simulink model "Inverse_v1"  (R2022a)
settings: Solver=VariableStepAuto  StartTime=0.0  StopTime=10.0  RelTol=1e-3
settings Model: Creator=maximilian  LastModifiedBy=maximilian

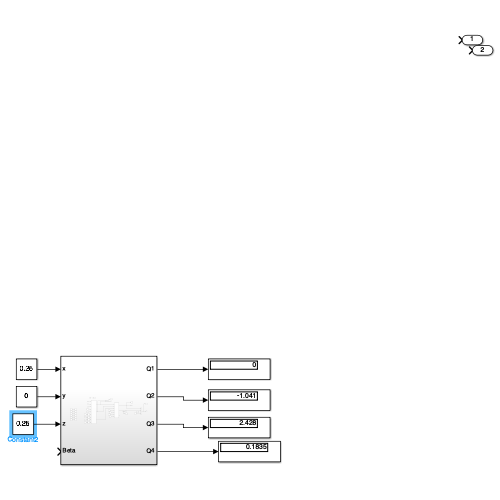
[thumbnail: Simulink's stored preview of the top-level diagram]
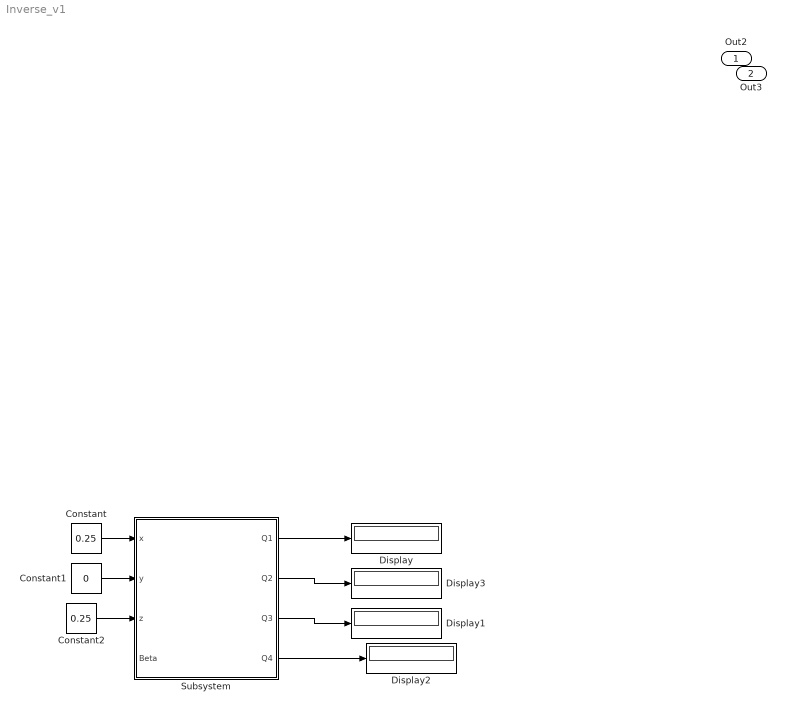
== system Inverse_v1 ==
  Constant : Constant  Value=0.25
  Constant1 : Constant  Value=0
  Constant2 : Constant  Value=0.25
  Display{,1..3} (4 alike) : Display
  Subsystem : Subsystem
  Out2 : Outport
  Out3 : Outport  Port=2
  wires:
  Constant2/1 -> Subsystem/3(z)
  Constant/1 -> Subsystem/1(x)
  Constant1/1 -> Subsystem/2(y)
  Subsystem/1(Q1) -> Display/1
  Subsystem/2(Q2) -> Display3/1
  Subsystem/3(Q3) -> Display1/1
  Subsystem/4(Q4) -> Display2/1

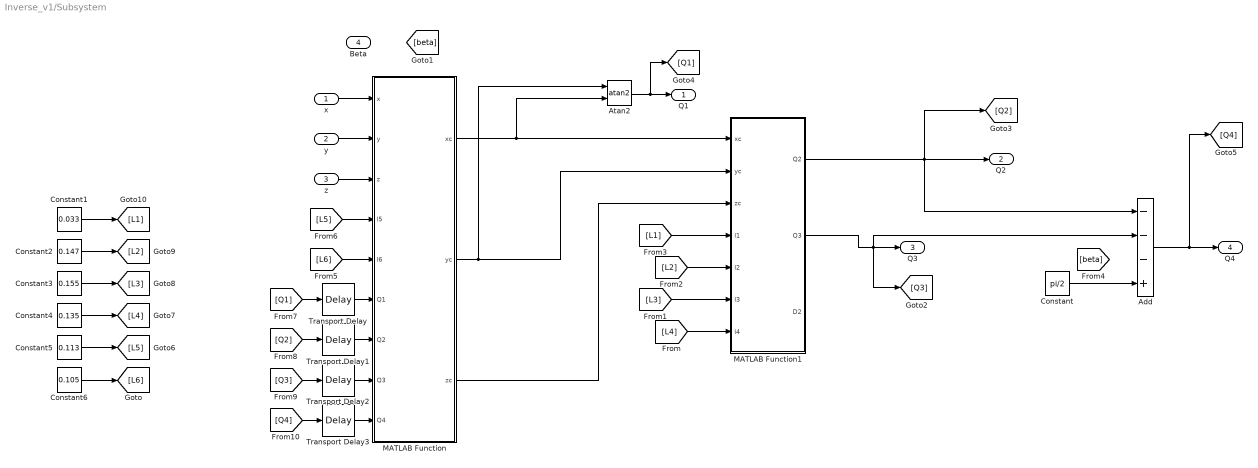
== system Inverse_v1/Subsystem ==
  x : Inport
  y : Inport  Port=2
  z : Inport  Port=3
  Beta : Inport  Port=4
  Add : Sum  Inputs=---+
  Atan2 : Trigonometry  Operator=atan2
  Constant : Constant  Value=pi/2
  Constant1 : Constant  Value=0.033
  Constant2 : Constant  Value=0.147
  Constant3 : Constant  Value=0.155
  Constant4 : Constant  Value=0.135
  Constant5 : Constant  Value=0.113
  Constant6 : Constant  Value=0.105
  MATLAB Function : MATLAB Function  TreatAsAtomicUnit=on
  MATLAB Function1 : MATLAB Function  TreatAsAtomicUnit=on
  Transport Delay{,1..3} (4 alike) : TransportDelay
  Q1 : Outport
  Q2 : Outport  Port=2
  Q3 : Outport  Port=3
  Q4 : Outport  Port=4
  wires:
  MATLAB Function/3(zc) -> MATLAB Function1/3(zc)
  Constant2/1 -> [L2]
  MATLAB Function/2(yc) -> Atan2/1, MATLAB Function1/2(yc)
  [L2] -> MATLAB Function1/5(l2)
  MATLAB Function1/2(Q3) -> Add/2, Q3/1, [Q3]
  Constant/1 -> Add/4
  [L3] -> MATLAB Function1/6(l3)
  [Q1] -> Transport Delay/1
  [Q4] -> Transport Delay3/1
  Transport Delay2/1 -> MATLAB Function/8(Q3)
  Transport Delay/1 -> MATLAB Function/6(Q1)
  [L1] -> MATLAB Function1/4(l1)
  [L5] -> MATLAB Function/4(l5)
  Transport Delay1/1 -> MATLAB Function/7(Q2)
  Constant1/1 -> [L1]
  Add/1 -> [Q4], Q4/1
  Atan2/1 -> Q1/1, [Q1]
  z/1 -> MATLAB Function/3(z)
  [Q3] -> Transport Delay2/1
  MATLAB Function/1(xc) -> MATLAB Function1/1(xc), Atan2/2
  x/1 -> MATLAB Function/1(x)
  [L4] -> MATLAB Function1/7(l4)
  MATLAB Function1/1(Q2) -> Add/1, Q2/1, [Q2]
  Transport Delay3/1 -> MATLAB Function/9(Q4)
  y/1 -> MATLAB Function/2(y)
  [L6] -> MATLAB Function/5(l6)
  [Q2] -> Transport Delay1/1
  Constant4/1 -> [L4]
  Constant6/1 -> [L6]
  Constant3/1 -> [L3]
  Constant5/1 -> [L5]

== matlab function Inverse_v1/Subsystem/MATLAB Function ==
  data: x input; xc output; y input; z input; l5 input; l6 input; Q1 input; Q2 input; Q3 input; Q4 input; yc output; zc output
function [xc, yc,zc] = Findoc(x,y,z,l5,l6,Q1,Q2,Q3,Q4)
 
 r13 = cos (Q1) *sin (Q2 + Q3 + Q4);
 r23 = sin (Q1) *sin (Q2 + Q3 + Q4);
 r33 = cos (Q2 + Q3 + Q4) ;

 xc=x - (l5+l6)*r13;
 yc = y - (l5+l6)*r23;
 zc = z - (l5+l6)*r33;

end

== matlab function Inverse_v1/Subsystem/MATLAB Function1 ==
  data: xc input; Q2 output; yc input; zc input; l1 input; l2 input; l3 input; l4 input; Q3 output; D2 output
function [Q2,Q3,D2] = fcn(xc,yc,zc,l1,l2,l3,l4)
D = ((xc^2+yc^2 - 2*sqrt(xc^2+yc^2)*l1 + l1^2)+(zc-l2)^2 - l3^2-l4^2)/(2*l3*l4);
D2 = 1 - D^2;
    if D2 < 0;
        Q3 = 0;
        Q2 = 0;
    else
        Q3 = atan2(sqrt(1-D^2),D);
        Q2 = atan2((sqrt(xc^2+yc^2)-l1),zc-l2) - atan2(l4*sin(Q3),l3+l4*cos(Q3));
    end

end
